simulink model "lab1"  (R2025b)
settings: Solver=VariableStepAuto  StartTime=0.0  StopTime=0.3  RelTol=1e-3
model workspace (MAT data in the model file):
  J = 3.2284e-06
  K = 0.0274
  Kd = 0.0005
  Ki = 1
  Kp = 0.5
  L = 2.75e-06
  R = 4
  b = 3.5077e-06
settings Model: Creator=banikt  LastModifiedBy=OWNER

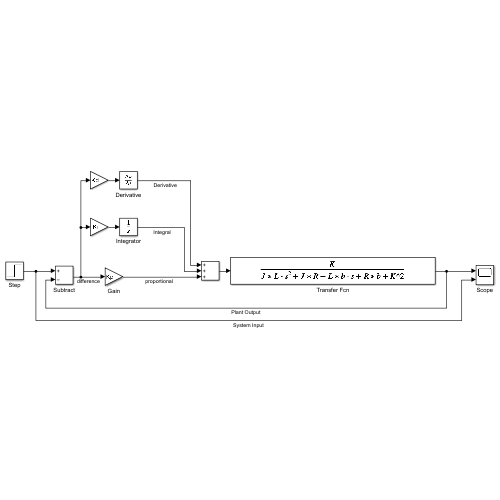
[thumbnail: Simulink's stored preview of the top-level diagram]
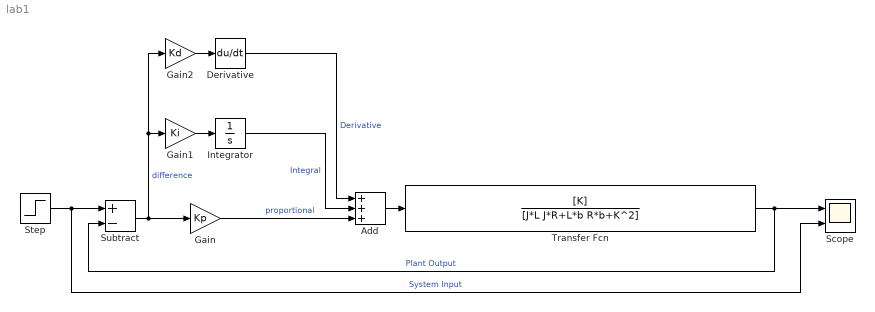
== system lab1 ==
  Add : Sum  Inputs=+++
  Derivative : Derivative
  Gain : Gain  Gain=Kp
  Gain1 : Gain  Gain=Ki
  Gain2 : Gain  Gain=Kd
  Integrator : Integrator
  Scope : Scope  NumInputPorts=2
      settings: ActiveDisplayYMinimum=-2.0179889619731739  ActiveDisplayYMaximum=62.040309784486652
  Step : Step  Time=0.01  After=60  SampleTime=0
  Subtract : Sum  Inputs=+-
  Transfer Fcn : TransferFcn  Numerator=[K]  Denominator=[J*L J*R+L*b R*b+K^2]
  wires:
  Step/1 -> Scope/2, Subtract/1  "System Input"
  Transfer Fcn/1 -> Subtract/2, Scope/1  "Plant Output"
  Subtract/1 -> Gain1/1, Gain2/1, Gain/1  "difference"
  Gain/1 -> Add/3  "proportional"
  Gain1/1 -> Integrator/1
  Add/1 -> Transfer Fcn/1
  Integrator/1 -> Add/2  "Integral"
  Derivative/1 -> Add/1  "Derivative"
  Gain2/1 -> Derivative/1
